simulink model "pns_priority"  (Simulink 8.8)
settings: Solver=ode45  StartTime=0  StopTime=20  RelTol=1e-3  EnableMultiTasking=on
values from neighbouring files (symbols this model uses):
  SubsystemMPC =     [agent.mat]
undefined symbols (not defined in the file or in its folder): Ac, Bc, Cc, Dc, HDMPC, hdmpc_control, Lc
settings Model: Creator=stefano  LastModifiedBy=trinhvv-admin
settings DataIOCC: SaveOutput=off  SignalLogging=off  DSMLogging=off  SaveTime=off
settings OptimizationCC: ExpressionDepthLimit=2147483647

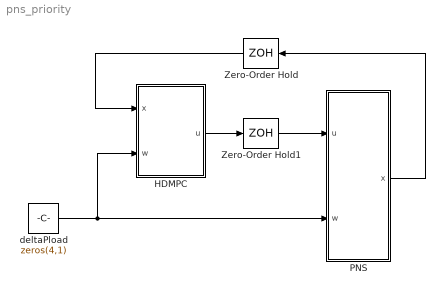
== system pns_priority ==
  HDMPC : Subsystem
  PNS : Subsystem
  Zero-Order Hold : ZeroOrderHold
  Zero-Order Hold1 : ZeroOrderHold
  deltaPload : Constant  Value=zeros(4,1)
  wires:
  PNS/1(x) -> Zero-Order Hold/1
  deltaPload/1 -> HDMPC/2(w), PNS/2(w)
  Zero-Order Hold/1 -> HDMPC/1(x)
  Zero-Order Hold1/1 -> PNS/1(u)
  HDMPC/1(u) -> Zero-Order Hold1/1

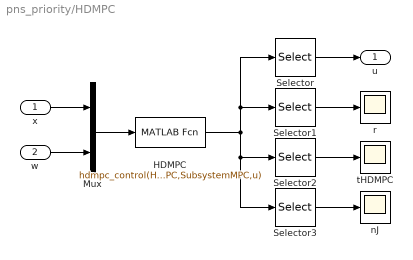
== system pns_priority/HDMPC ==
  x : Inport
  w : Inport  Port=2
  HDMPC : MATLABFcn  MATLABFcn=hdmpc_control(HDMPC,SubsystemMPC,u)  OutputDimensions=10
  Mux : Mux  Inputs=2
  Selector : Selector  IndexOptions=Index vector (dialog)  Indices=1:4  OutputSizes=1
  Selector1 : Selector  IndexOptions=Index vector (dialog)  Indices=5:8  OutputSizes=1
  Selector2 : Selector  IndexOptions=Index vector (dialog)  Indices=9  OutputSizes=1
  Selector3 : Selector  IndexOptions=Index vector (dialog)  Indices=10  OutputSizes=1
  nJ : Scope
  r : Scope
  tHDMPC : Scope
  u : Outport
  wires:
  Selector/1 -> u/1
  HDMPC/1 -> Selector3/1, Selector2/1, Selector/1, Selector1/1
  Mux/1 -> HDMPC/1
  x/1 -> Mux/1
  w/1 -> Mux/2
  Selector1/1 -> r/1
  Selector2/1 -> tHDMPC/1
  Selector3/1 -> nJ/1

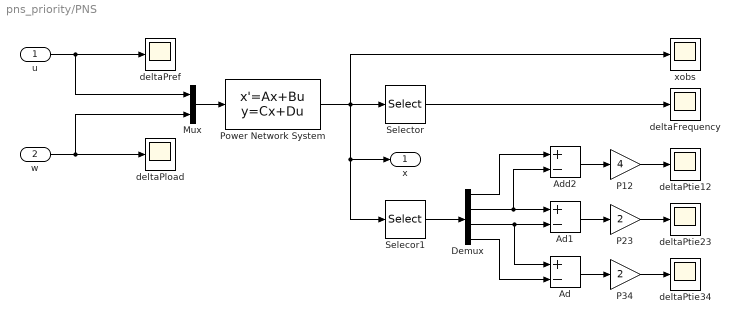
== system pns_priority/PNS ==
  u : Inport
  w : Inport  Port=2
  Ad : Sum  Inputs=+-
  Ad1 : Sum  Inputs=+-
  Add2 : Sum  Inputs=+-
  Demux : Demux
  Mux : Mux  Inputs=2
  P12 : Gain  Gain=4
  P23 : Gain  Gain=2
  P34 : Gain  Gain=2
  Power Network System : StateSpace  A=Ac  B=[ Bc Lc ]  C=Cc  D=[ Dc zeros(size(Cc,1),size(Lc,2)) ]  X0=|
      | [   -0.0297
      |     0.0662
      |     0.0171
      |     0.0099
      |     0.0834
      |    -0.0428
      |     0.0514
      |     0.0507
      |    -0.0239
      |     0.0136
      |    -0.0848
      |    -0.0892
      |     0.0062
      |     0.0558
      |     0.0868
      |    -0.0740]'
  Selecor1 : Selector  InputPortWidth=16  IndexOptions=Index vector (dialog)  Indices=1:4:size(Ac,1)  OutputSizes=1
  Selector : Selector  InputPortWidth=16  IndexOptions=Index vector (dialog)  Indices=2:4:size(Ac,1)  OutputSizes=1
  deltaFrequency : Scope
  deltaPload : Scope
  deltaPref : Scope
  deltaPtie12 : Scope
  deltaPtie23 : Scope
  deltaPtie34 : Scope
  xobs : Scope
  x : Outport
  wires:
  Power Network System/1 -> x/1, Selecor1/1, xobs/1, Selector/1
  Mux/1 -> Power Network System/1
  w/1 -> Mux/2, deltaPload/1
  u/1 -> Mux/1, deltaPref/1
  Selector/1 -> deltaFrequency/1
  Selecor1/1 -> Demux/1
  Add2/1 -> P12/1
  P12/1 -> deltaPtie12/1
  Ad1/1 -> P23/1
  P23/1 -> deltaPtie23/1
  Ad/1 -> P34/1
  P34/1 -> deltaPtie34/1
  Demux/1 -> Add2/1
  Demux/2 -> Ad1/1, Add2/2
  Demux/3 -> Ad1/2, Ad/1
  Demux/4 -> Ad/2
